simulink model "Controllo_inverso_RNE_RE_velocita"  (R2020a)
settings: Solver=daessc  StartTime=0.0  StopTime=run_time  FixedStep=0.01  MinStep=0.01  RelTol=1e-3
values from neighbouring files (symbols this model uses):
  T = [a,a,0,0;-a,a,0,0;0,0,1,0.1034;0,0,0,1]    [mdl_panda_RE.m]
undefined symbols (not defined in the file or in its folder): A, accel_panda_RNE_RE, controllo_interno_RNE_RE, ddqmax, dq0, dqmax, Kgain, panda_RE, q0, qmax2, qmin, run_time, velocita_sin
settings Model: Creator=bele  LastModifiedBy=gabri
settings DebuggingCC: SFMachineParentedDataDiag=error

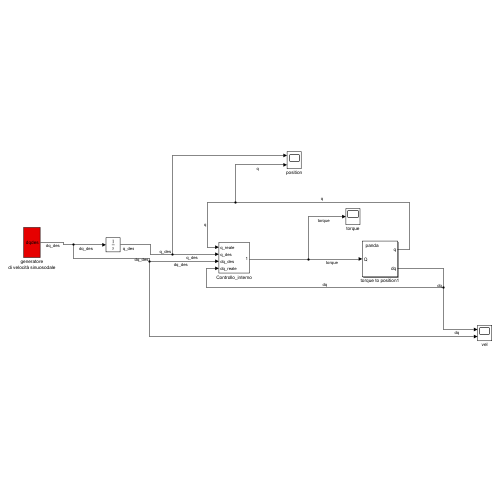
[thumbnail: Simulink's stored preview of the top-level diagram]
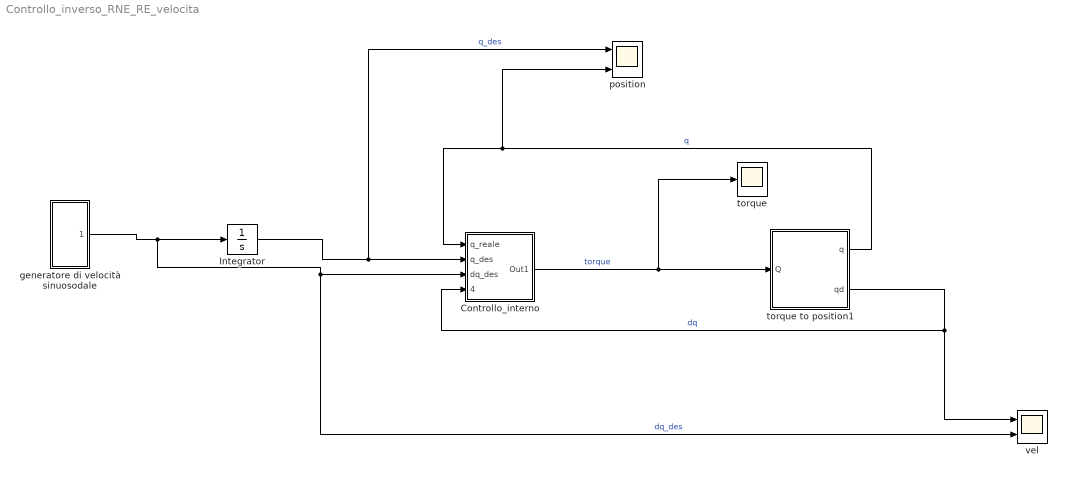
== system Controllo_inverso_RNE_RE_velocita ==
  Controllo_interno : Subsystem  mask{ddqmax=ddqmax, K=Kgain, dt=0.01, robot=panda_RE}
  Integrator : Integrator  InitialCondition=q0
  generatore di velocità sinuosodale : Subsystem  mask{dqmax=dqmax, A=A, run_time=run_time, T=T}
      mask help: Joint interpolated trajectory.
      mask init:
      | t=[0:100]'/100*run_time;
      mask Help:
      | Generate quintic polynomial to move from initial to final joint angles as specified.  Initial and final velocity are assumed to be zero.
      | 
      | <b>Parameters::</b>
      | 
      | q0 (1xN) initial joint coordinates
      | qf (1xN) final joint coordinates
      | tmax (1x1) the time for the trajectory to complete
      | 
      | Initial and final velocity are assumed to be zero.
      | 
      | <b>Outputs::</b>
      | 
      | q (1xN) vector of joint coordinates at current simulation time
      | qd (1xN) vector of joint coordinate velocity at current simulation time
      | qdd (1xN) vector of joint coordinate acceleration at current simulation time
      | 
      | <b>Notes::</b>
      | 
      | - If simulation time exceeds tmax then q is clipped to qf.
      | - A wrapper on the Toolbox function jtraj.
      | - The piecewise constant output of jtraj is interpolated to the current
      |   simulation time.
      mask Display: port_label('output', 1, 'dqdes')
  position : Scope  NumInputPorts=2
  torque : Scope
  torque to position1 : Subsystem  mask{q0=q0, dq0=dq0, robot=panda_RE}
      mask prompts: q0 "Initial state"
      mask help: Rigid-body dynamic model of robot.
      mask init:
      | rname = 'panda';
      | n = 7;
      mask Help:
      | Simulates the forward (direct) rigid-body dynamics of the robot described
      | by the given robot object.  For given applied joint torque/force it computes
      | the instaneous joint coordinates, velocities and acclerations.
      | 
      | 
      | <b>Parameters::</b>
      | 
      | robot (SerialLink) a dynamic model of an N-link serial link manipulator
      | q0 (1xN)  Initial joint coordinates
      | 
      | <b>Inputs::</b>
      | 
      | Q (1xN) the generalized joint force (torque or force) required to achieve
      | the motion state (q, qd, qdd).
      | 
      | <b>Outputs::</b>
      | 
      | q (1xN) joint coordinates
      | qd (1xN) joint coordinate velocity
      | qdd (1xN) joint coordinate acceleration
      | 
      | 
      | <b>Notes::</b>
      | 
      | - Required to simulate robot rigid body motion.
      | - Implemented using the recursive Newton-Euler scheme (RNE).
      | - A wrapper for the Toolbox method accel() which in turn depends on the
      |   method rne().
      mask Display:
      | port_label('input', 1, 'Q')
      | port_label('output', 1, 'q')
      | port_label('output', 2, 'dq')
      | text(0.1, 0.9,  rname, 'horizontalAlignment', 'left')
  vel : Scope  NumInputPorts=2
  wires:
  generatore di velocità sinuosodale/1(q_des) -> vel/2, Controllo_interno/3(dq_des), Integrator/1  "dq_des"
  torque to position1/1(q) -> position/2, Controllo_interno/1(q_reale)  "q"
  Integrator/1 -> position/1, Controllo_interno/2(q_des)  "q_des"
  torque to position1/2(qd) -> vel/1, Controllo_interno/4(dq_reale)  "dq"
  Controllo_interno/1(Out1) -> torque/1, torque to position1/1(Q)  "torque"

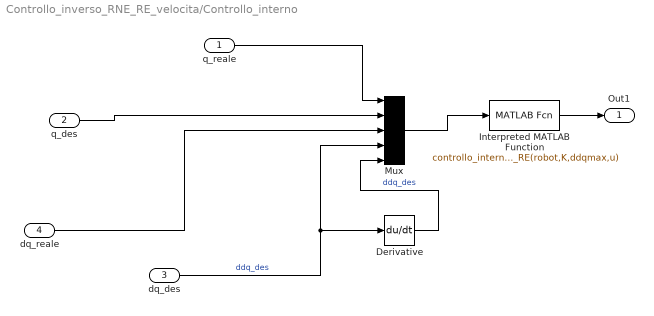
== system Controllo_inverso_RNE_RE_velocita/Controllo_interno ==
  q_reale : Inport
  q_des : Inport  Port=2
  dq_des : Inport  Port=3
  dq_reale : Inport  Port=4
  Derivative : Derivative
  Interpreted MATLAB Function : MATLABFcn  MATLABFcn=controllo_interno_RNE_RE(robot,K,ddqmax,u)
  Mux : Mux  Inputs=5
  Out1 : Outport
  wires:
  Interpreted MATLAB Function/1 -> Out1/1
  Mux/1 -> Interpreted MATLAB Function/1
  dq_reale/1 -> Mux/3
  q_reale/1 -> Mux/1
  q_des/1 -> Mux/2
  dq_des/1 -> Derivative/1, Mux/4  "ddq_des"
  Derivative/1 -> Mux/5  "ddq_des"

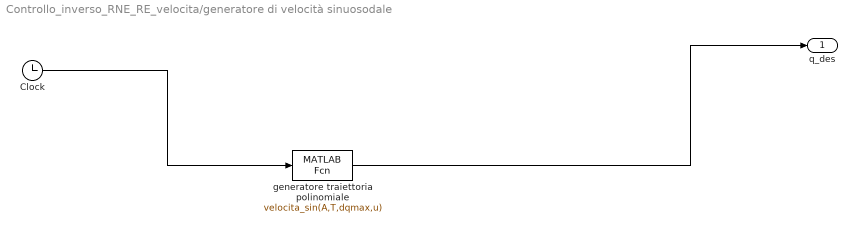
== system Controllo_inverso_RNE_RE_velocita/generatore di velocità sinuosodale ==
  Clock : Clock
  generatore traiettoria polinomiale : MATLABFcn  MATLABFcn=velocita_sin(A,T,dqmax,u)
  q_des : Outport  VectorParamsAs1DForOutWhenUnconnected=off
  wires:
  generatore traiettoria polinomiale/1 -> q_des/1
  Clock/1 -> generatore traiettoria polinomiale/1

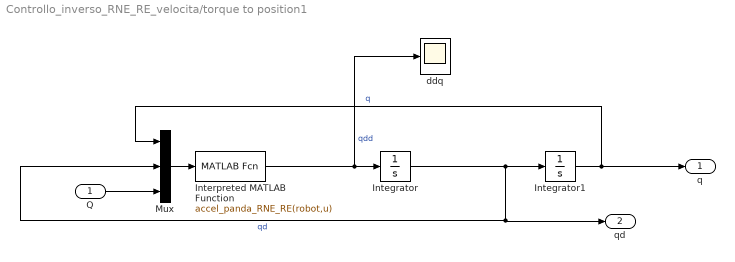
== system Controllo_inverso_RNE_RE_velocita/torque to position1 ==
  Q : Inport
  Integrator : Integrator  InitialCondition=dq0  UpperSaturationLimit=dqmax  LowerSaturationLimit=-dqmax
  Integrator1 : Integrator  InitialCondition=q0  UpperSaturationLimit=qmax2  LowerSaturationLimit=qmin
  Interpreted MATLAB Function : MATLABFcn  MATLABFcn=accel_panda_RNE_RE(robot,u)
  Mux : Mux  Inputs=3
  ddq : Scope
  q : Outport  VectorParamsAs1DForOutWhenUnconnected=off
  qd : Outport  Port=2  VectorParamsAs1DForOutWhenUnconnected=off
  wires:
  Integrator1/1 -> q/1, Mux/1  "q"
  Interpreted MATLAB Function/1 -> ddq/1, Integrator/1  "qdd"
  Mux/1 -> Interpreted MATLAB Function/1
  Integrator/1 -> Integrator1/1, Mux/2, qd/1  "qd"
  Q/1 -> Mux/3
